simulink library "untitled1"  (R2023b)
settings: Solver=VariableStepAuto  StartTime=0.0  StopTime=10.0  RelTol=1e-3
undefined symbols (not defined in the file): C, R
settings Model: Creator=mueller.chris-it22  LastModifiedBy=mueller.chris-it22

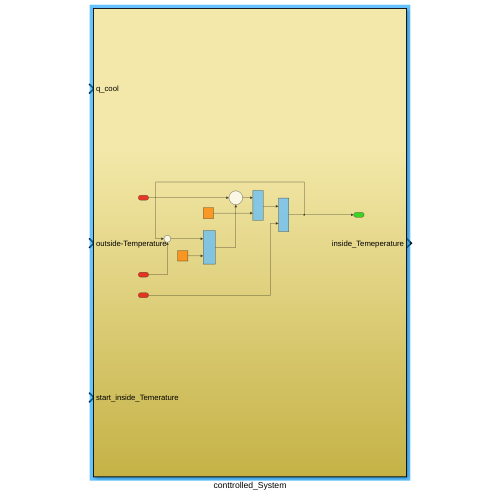
[thumbnail: Simulink's stored preview of the top-level diagram]
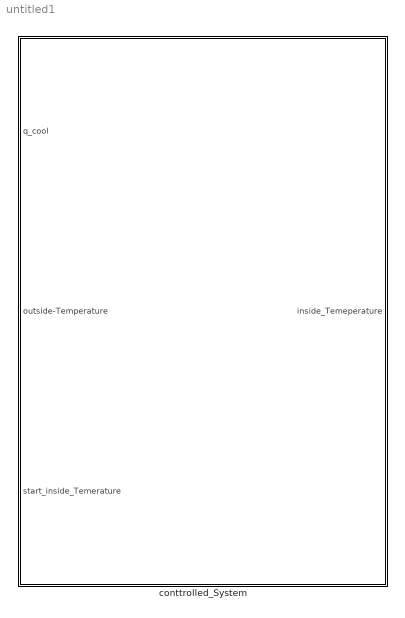
== system untitled1 ==
  conttrolled_System : Subsystem

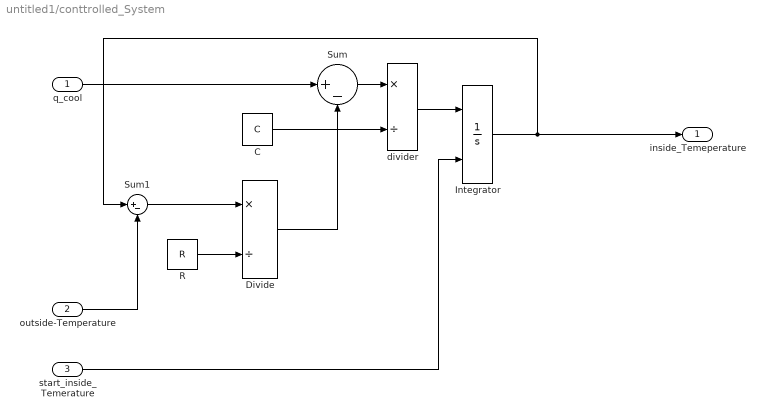
== system untitled1/conttrolled_System ==
  q_cool : Inport
  outside-Temperature : Inport  Port=2
  start_inside_Temerature : Inport  Port=3
  C : Constant  Value=C
  Divide : Product  Inputs=*/
  Integrator : Integrator  InitialConditionSource=external
  R : Constant  Value=R
  Sum : Sum  Inputs=|+-
  Sum1 : Sum  Inputs=|+-
  divider : Product  Inputs=*/
  inside_Temeperature : Outport
  wires:
  Sum/1 -> divider/1
  Sum1/1 -> Divide/1
  divider/1 -> Integrator/1
  R/1 -> Divide/2
  C/1 -> divider/2
  q_cool/1 -> Sum/1
  Divide/1 -> Sum/2
  outside-Temperature/1 -> Sum1/2
  Integrator/1 -> Sum1/1, inside_Temeperature/1
  start_inside_Temerature/1 -> Integrator/2
